simulink library "ayazPlant_cl"  (R2018b)
settings: Solver=VariableStepAuto  StartTime=0.0  StopTime=10.0  RelTol=1e-3
undefined symbols (not defined in the file or in its folder): sim_param
libraries: ayazLiftingBody_cl x1, ayazTethers_cl x1, ayazWinches_cl x1, threeTetherGroundStation_cl x1
settings Model: Creator=mcobb  LastModifiedBy=mcobb

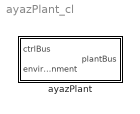
== system ayazPlant_cl ==
  ayazPlant : Subsystem

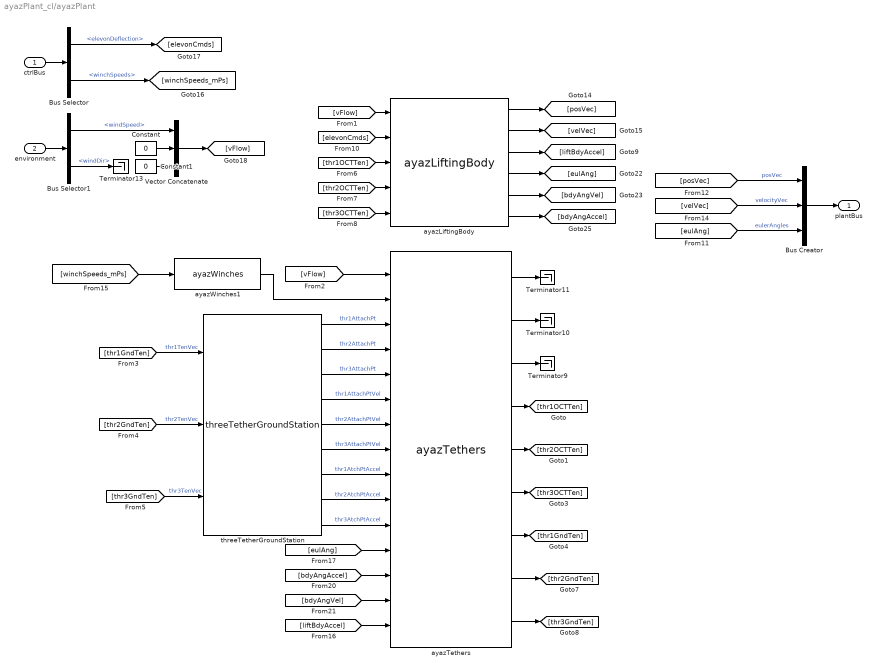
== system ayazPlant_cl/ayazPlant ==
  ctrlBus : Inport  OutDataTypeStr=Bus: ctrlBus
  environment : Inport  Port=2  OutDataTypeStr=Bus: envBus
  Bus Creator : BusCreator  Inputs=3  OutDataTypeStr=Bus: plantBus
  Bus Selector : BusSelector  OutputSignals=elevonDeflection,winchSpeeds
  Bus Selector1 : BusSelector  OutputSignals=windSpeed,windDir
  Constant : Constant  Value=0
  Constant1 : Constant  Value=0
  Terminator{9..11,13} (4 alike) : Terminator
  Vector Concatenate : Concatenate  NumInputs=3
  ayazLiftingBody : ayazLiftingBody_cl/ayazLiftingBody  SystemSampleTime=-1
  ayazTethers : ayazTethers_cl/ayazTethers  SystemSampleTime=-1
  ayazWinches1 : ayazWinches_cl/ayazWinches  SystemSampleTime=-1
  threeTetherGroundStation : threeTetherGroundStation_cl/threeTetherGroundStation  fixed=1  J=sim_param.platform_param.platform_Izz  b=sim_param.platform_param.platform_damping  posVec=[0 0 0]  thr1AttachPt=sim_param.tether_imp_nodes.R11_g  thr2AttachPt=sim_param.tether_imp_nodes.R21_g  thr3AttachPt=sim_param.tether_imp_nodes.R31_g  initAngPos=ini_platform_ang  initAngVel=ini_platform_vel
  plantBus : Outport  OutDataTypeStr=Bus: plantBus
  wires:
  ayazTethers/4 -> [thr1OCTTen]
  ayazTethers/6 -> [thr3OCTTen]
  ayazTethers/5 -> [thr2OCTTen]
  ayazTethers/7 -> [thr1GndTen]
  ayazTethers/8 -> [thr2GndTen]
  ayazTethers/9 -> [thr3GndTen]
  ayazTethers/3 -> Terminator9/1
  ayazTethers/2 -> Terminator10/1
  ayazTethers/1 -> Terminator11/1
  ayazWinches1/1 -> ayazTethers/2
  ayazLiftingBody/3 -> [liftBdyAccel]
  ayazLiftingBody/4 -> [eulAng]
  ayazLiftingBody/1 -> [posVec]
  ayazLiftingBody/2 -> [velVec]
  [vFlow] -> ayazTethers/1
  [vFlow] -> ayazLiftingBody/1
  [thr1OCTTen] -> ayazLiftingBody/3
  [thr2OCTTen] -> ayazLiftingBody/4
  [thr3OCTTen] -> ayazLiftingBody/5
  [winchSpeeds_mPs] -> ayazWinches1/1
  [elevonCmds] -> ayazLiftingBody/2
  environment/1 -> Bus Selector1/1
  ctrlBus/1 -> Bus Selector/1
  Bus Selector1/2 -> Terminator13/1  "<windDir>"
  Bus Selector/1 -> [elevonCmds]  "<elevonDeflection>"
  Bus Selector1/1 -> Vector Concatenate/1  "<windSpeed>"
  Bus Selector/2 -> [winchSpeeds_mPs]  "<winchSpeeds>"
  Bus Creator/1 -> plantBus/1
  [posVec] -> Bus Creator/1  "posVec"
  [eulAng] -> Bus Creator/3  "eulerAngles"
  [velVec] -> Bus Creator/2  "velocityVec"
  Vector Concatenate/1 -> [vFlow]
  Constant/1 -> Vector Concatenate/2
  Constant1/1 -> Vector Concatenate/3
  ayazLiftingBody/5 -> [bdyAngVel]
  ayazLiftingBody/6 -> [bdyAngAccel]
  [thr3GndTen] -> threeTetherGroundStation/3  "thr3TenVec"
  [thr2GndTen] -> threeTetherGroundStation/2  "thr2TenVec"
  [thr1GndTen] -> threeTetherGroundStation/1  "thr1TenVec"
  [liftBdyAccel] -> ayazTethers/15
  [bdyAngVel] -> ayazTethers/14
  [bdyAngAccel] -> ayazTethers/13
  [eulAng] -> ayazTethers/12
  threeTetherGroundStation/1 -> ayazTethers/3  "thr1AttachPt"
  threeTetherGroundStation/2 -> ayazTethers/4  "thr2AttachPt"
  threeTetherGroundStation/3 -> ayazTethers/5  "thr3AttachPt"
  threeTetherGroundStation/4 -> ayazTethers/6  "thr1AttachPtVel"
  threeTetherGroundStation/5 -> ayazTethers/7  "thr2AttachPtVel"
  threeTetherGroundStation/6 -> ayazTethers/8  "thr3AttachPtVel"
  threeTetherGroundStation/7 -> ayazTethers/9  "thr1AtchPtAccel"
  threeTetherGroundStation/8 -> ayazTethers/10  "thr2AtchPtAccel"
  threeTetherGroundStation/9 -> ayazTethers/11  "thr3AtchPtAccel"
